simulink model "sensors"  (R2025b)
settings: Solver=FixedStepAuto  StartTime=0.0  StopTime=10.0  RelTol=1e-3
undefined symbols (not defined in the file): g, imu, mocap
libraries: aerolibutil x3, sharedutil x2, aerolibnav x2
settings Model: DataDictionary=project.sldd  Creator=Nick  LastModifiedBy=Nick

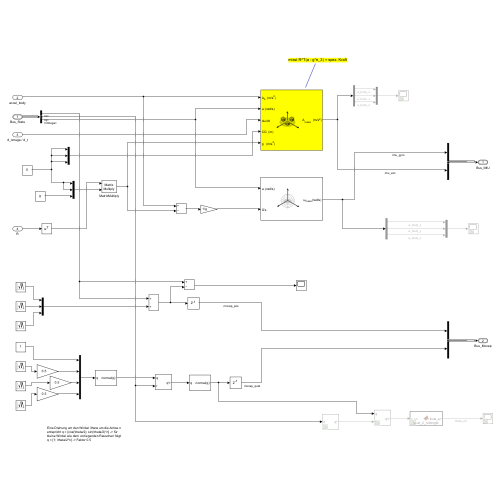
[thumbnail: Simulink's stored preview of the top-level diagram]
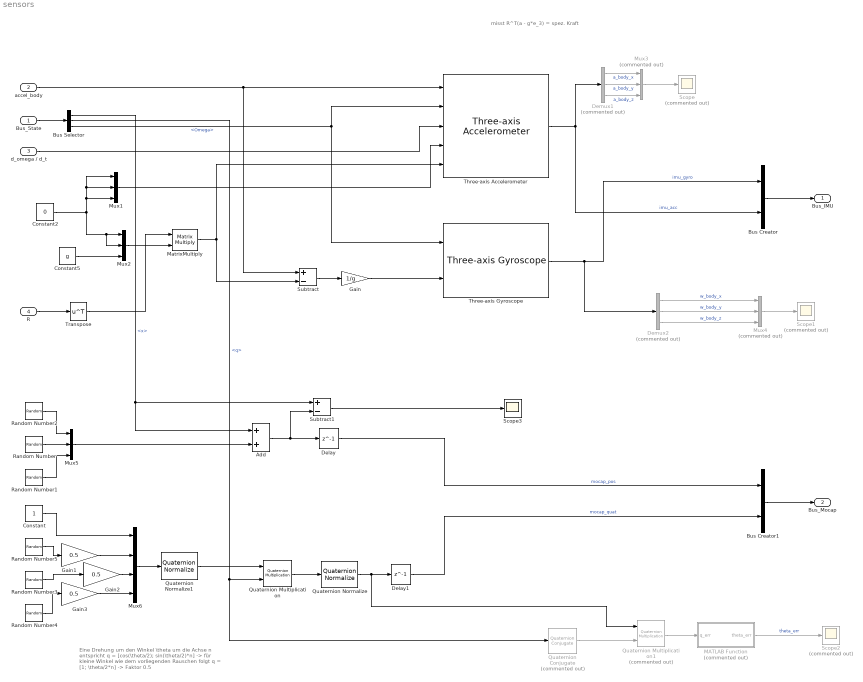
== system sensors ==
  note: misst R^T(a - g*e_3) = spez. Kraft
  note: Eine Drehung um den Winkel \theta um die Achse n
      | entspricht q = [cos(\theta/2); sin(\theta/2)*n] -> für
      | kleine Winkel wie dem vorliegenden Rauschen folgt
      | q = [1; \theta/2*n] -> Faktor 0.5
  Bus_State : Inport  OutDataTypeStr=Bus: Bus_State
  accel_body : Inport  Port=2
  d_omega / d_t : Inport  Port=3
  R : Inport  Port=4  PortDimensions=[3,3]
  Add : Sum
  Bus Creator : BusCreator  Inputs=2  OutDataTypeStr=Bus: Bus_IMU  NonVirtualBus=on
  Bus Creator1 : BusCreator  Inputs=2  OutDataTypeStr=Bus: Bus_Mocap  NonVirtualBus=on
  Bus Selector : BusSelector  OutputSignals=x,q,Omega
  Constant : Constant
  Constant2 : Constant  Value=0
  Constant5 : Constant  Value=g
  Delay : Delay  DelayLength=1  SampleTime=mocap.Ts_mocap
  Delay1 : Delay  DelayLength=1  SampleTime=mocap.Ts_mocap
  Demux1 : Demux  Commented=on  Outputs=3
  Demux2 : Demux  Commented=on  Outputs=3
  Gain : Gain  Gain=1/g
  Gain1 : Gain  Gain=0.5
  Gain2 : Gain  Gain=0.5
  Gain3 : Gain  Gain=0.5
  MATLAB Function : MATLAB Function  Commented=on  TreatAsAtomicUnit=on
  MatrixMultiply : Product  Multiplication=Matrix(*)
  Mux1 : Mux  Inputs=3
  Mux2 : Mux  Inputs=3
  Mux3 : Mux  Commented=on  Inputs=3
  Mux4 : Mux  Commented=on  Inputs=3
  Mux5 : Mux  Inputs=3
  Mux6 : Mux
  Quaternion Conjugate : aerolibutil/Quaternion Conjugate  Commented=on
  Quaternion Multiplication : aerolibutil/Quaternion Multiplication
  Quaternion Multiplication1 : aerolibutil/Quaternion Multiplication  Commented=on
  Quaternion Normalize : sharedutil/Quaternion Normalize  aMode=aMode
  Quaternion Normalize1 : sharedutil/Quaternion Normalize  aMode=aMode
  Random Number : RandomNumber  Variance=mocap.pos_noise^2  Seed=1  SampleTime=mocap.Ts_mocap
  Random Number1 : RandomNumber  Variance=mocap.pos_noise^2  Seed=2  SampleTime=mocap.Ts_mocap
  Random Number2 : RandomNumber  Variance=mocap.pos_noise^2  SampleTime=mocap.Ts_mocap
  Random Number3 : RandomNumber  Variance=mocap.att_noise^2  Seed=4  SampleTime=mocap.Ts_mocap
  Random Number4 : RandomNumber  Variance=mocap.att_noise^2  Seed=5  SampleTime=mocap.Ts_mocap
  Random Number5 : RandomNumber  Variance=mocap.att_noise^2  Seed=3  SampleTime=mocap.Ts_mocap
  Scope : Scope  Commented=on
      settings: ActiveDisplayYMinimum=-12.218115911267493  ActiveDisplayYMaximum=2.2394488753574371
  Scope1 : Scope  Commented=on
      settings: ActiveDisplayYMinimum=-1  ActiveDisplayYMaximum=1
  Scope2 : Scope  Commented=on
      settings: ActiveDisplayYMinimum=-0.0045196791612787191  ActiveDisplayYMaximum=0.049921461821229356  DataLoggingVariableName=ScopeData2
  Scope3 : Scope
      settings: ActiveDisplayYMinimum=-1  ActiveDisplayYMaximum=1  DataLoggingVariableName=ScopeData3
  Subtract : Sum  Inputs=+-
  Subtract1 : Sum  Inputs=+-
  Three-axis Accelerometer : aerolibnav/Three-axis Accelerometer  units=Metric (MKS)  acc=[0 0 0]  gtype=on  dtype_a=on  w_a=imu.acc_wn  z_a=imu.acc_zeta  a_sf_cc=imu.acc_M  a_bias=imu.acc_bias  a_Ts=imu.Ts  a_rand=on  a_seeds=[23093 23094 23095]  a_pow=imu.acc_PSD*[1 1 1]  a_sat="imu.acc_FSR*[-1  -1  -1  1 1 1]"
  Three-axis Gyroscope : aerolibnav/Three-axis Gyroscope  dtype_g=on  w_g=imu.gyro_wn  z_g=imu.gyro_zeta  g_sf_cc=imu.gyro_M  g_bias=imu.gyro_bias  g_sen=imu.gyro_gsens  g_Ts=imu.Ts  g_rand=on  g_seeds=[23093 23094 23095]  g_pow=imu.gyro_PSD*[1 1 1]  g_sat="imu.gyro_FSR*[-1  -1  -1  1 1 1]"
  Transpose : Math  Operator=transpose
  Bus_IMU : Outport  OutDataTypeStr=Bus: Bus_IMU
  Bus_Mocap : Outport  Port=2  OutDataTypeStr=Bus: Bus_Mocap
  wires:
  accel_body/1 -> Subtract/1, Three-axis Accelerometer/1
  Constant5/1 -> Mux2/3
  d_omega / d_t/1 -> Three-axis Accelerometer/3
  Constant2/1 -> Mux2/2, Mux2/1, Mux1/3, Mux1/2, Mux1/1
  Mux1/1 -> Three-axis Accelerometer/4
  Three-axis Accelerometer/1 -> Demux1/1, Bus Creator/2  "imu_acc"
  Demux1/1 -> Mux3/1  "a_body_x"
  Demux1/2 -> Mux3/2  "a_body_y"
  Demux1/3 -> Mux3/3  "a_body_z"
  Mux3/1 -> Scope/1
  Mux2/1 -> MatrixMultiply/2
  R/1 -> Transpose/1
  MatrixMultiply/1 -> Three-axis Accelerometer/5, Subtract/2
  Subtract/1 -> Gain/1
  Bus Creator/1 -> Bus_IMU/1
  Gain/1 -> Three-axis Gyroscope/2
  Demux2/3 -> Mux4/3  "w_body_z"
  Three-axis Gyroscope/1 -> Bus Creator/1, Demux2/1  "imu_gyro"
  Mux4/1 -> Scope1/1
  Demux2/1 -> Mux4/1  "w_body_x"
  Demux2/2 -> Mux4/2  "w_body_y"
  Add/1 -> Subtract1/2, Delay/1
  Delay/1 -> Bus Creator1/1  "mocap_pos"
  Random Number/1 -> Mux5/2
  Random Number2/1 -> Mux5/1
  Random Number1/1 -> Mux5/3
  Mux5/1 -> Add/2
  Random Number5/1 -> Gain1/1
  Random Number3/1 -> Gain2/1
  Constant/1 -> Mux6/1
  Quaternion Normalize1/1 -> Quaternion Multiplication/1
  Quaternion Multiplication/1 -> Quaternion Normalize/1
  Quaternion Normalize/1 -> Quaternion Multiplication1/1, Delay1/1
  Delay1/1 -> Bus Creator1/2  "mocap_quat"
  Mux6/1 -> Quaternion Normalize1/1
  Gain1/1 -> Mux6/2
  Gain2/1 -> Mux6/3
  Gain3/1 -> Mux6/4
  Random Number4/1 -> Gain3/1
  Quaternion Conjugate/1 -> Quaternion Multiplication1/2
  Quaternion Multiplication1/1 -> MATLAB Function/1(q_err)
  MATLAB Function/1(theta_err) -> Scope2/1  "theta_err"
  Bus Creator1/1 -> Bus_Mocap/1
  Subtract1/1 -> Scope3/1
  Bus_State/1 -> Bus Selector/1
  Bus Selector/3 -> Three-axis Accelerometer/2, Three-axis Gyroscope/1  "<Omega>"
  Bus Selector/1 -> Add/1, Subtract1/1  "<x>"
  Bus Selector/2 -> Quaternion Multiplication/2, Quaternion Conjugate/1  "<q>"
  Transpose/1 -> MatrixMultiply/1

== matlab function sensors/MATLAB Function ==
  data: q_err input; theta_err output
function theta_err = quat_2_rotAngle(q_err)   %#codegen
    theta_err = 2*atan2(norm(q_err(2:4)), abs(q_err(1)));
end
